simulink model "F16_Simulink_doublet"  (R2013b)
settings: Solver=ode4  StartTime=0.0  StopTime=50  FixedStep=0.01  RelTol=1e-3
InitFcn:
  | close all; clear; clc;
  | 
  | % Carrega as pastas do sistema
  | MainPath = pwd;
  | Folders = {'Turbina'; 'Atmosfera'; 'Modelo';
  |                  'CoeficientesAerodinamicos'};
  | 
  | for i = 1:numel(Folders)
  |     Pasta = [MainPath '/' Folders{i}];
  |     rmpath(Pasta);
  |     addpath(Pasta);
  | end
  | 
  | % Carrega os valores trimados.
  | load('Trimados.mat');
  | 
  | x0 = x;
values from neighbouring files (symbols this model uses):
  x = [502 0.0370186488564 2.59604154662e-07 0 0.0370186488564 0 0 0 0 0 0 0 ... (13 elements, 1x13)]    [Trimados.mat]
settings Model: Creator=Eduardo  LastModifiedBy=Eduardo

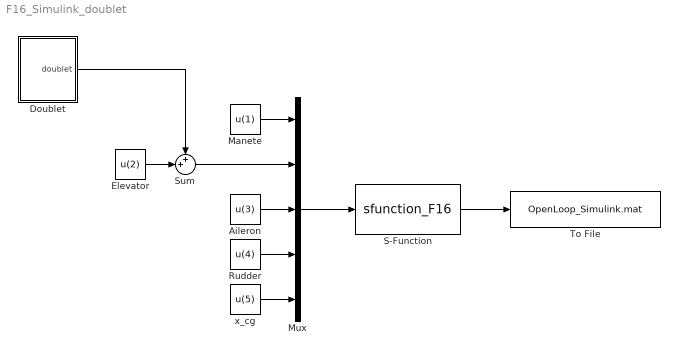
== system F16_Simulink_doublet ==
  Aileron : Constant  Value=u(3)
  Doublet : Subsystem
  Elevator : Constant  Value=u(2)
  Manete : Constant  Value=u(1)
  Mux : Mux  Inputs=5
  Rudder : Constant  Value=u(4)
  S-Function : S-Function  FunctionName=sfunction_F16  Parameters=x0  EnableBusSupport=off
  Sum : Sum  Inputs=++|
  To File : ToFile  Filename=OpenLoop_Simulink.mat  SampleTime=0.01
  x_cg : Constant  Value=u(5)
  wires:
  S-Function/1 -> To File/1
  Rudder/1 -> Mux/4
  Aileron/1 -> Mux/3
  x_cg/1 -> Mux/5
  Manete/1 -> Mux/1
  Mux/1 -> S-Function/1
  Elevator/1 -> Sum/2
  Sum/1 -> Mux/2
  Doublet/1(doublet) -> Sum/1

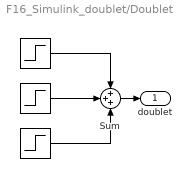
== system F16_Simulink_doublet/Doublet ==
  " " : Step  SampleTime=0
  "  " : Step  Time=1.5  After=-2  SampleTime=0
  "   " : Step  Time=2  SampleTime=0
  Sum : Sum  Inputs=+++
  doublet : Outport
  wires:
  " "/1 -> Sum/1
  "  "/1 -> Sum/2
  "   "/1 -> Sum/3
  Sum/1 -> doublet/1
